simulink model "AM"  (R2020a)
settings: Solver=VariableStepAuto  StartTime=0.0  StopTime=10.0  RelTol=1e-3
libraries: dsparch4 x1
settings Model: Creator=Admin  LastModifiedBy=fazal
settings SFSimCC: CustomCodeUndefinedFunction=UseInterfaceOnly

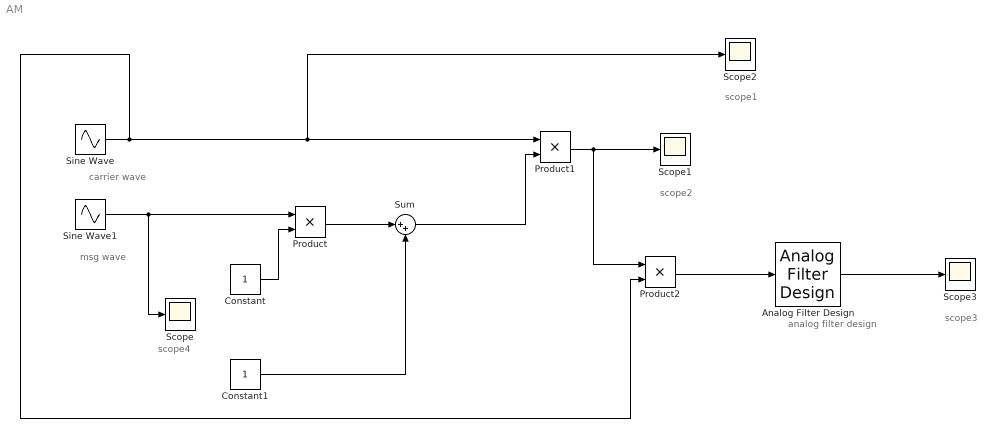
== system AM ==
  note: scope3
  note: scope1
  note: scope2
  note: scope4
  note: analog filter design
  note: msg wave
  note: carrier wave
  Analog Filter Design : dsparch4/Analog Filter Design  method=Butterworth  filttype=Lowpass  N=8  Wlo=30  Whi=80  Rp=2  Rs=40
  Constant : Constant
  Constant1 : Constant
  Product : Product
  Product1 : Product
  Product2 : Product
  Scope{,1..3} (4 alike) : Scope
  Sine Wave : Sin  Amplitude=2  Frequency=2*pi*5  SampleTime=0
  Sine Wave1 : Sin  Frequency=2*pi*1  SampleTime=0
  Sum : Sum  Inputs=|++
  wires:
  Product2/1 -> Analog Filter Design/1
  Analog Filter Design/1 -> Scope3/1
  Sum/1 -> Product1/2
  Product1/1 -> Product2/1, Scope1/1
  Sine Wave1/1 -> Scope/1, Product/1
  Constant/1 -> Product/2
  Product/1 -> Sum/1
  Constant1/1 -> Sum/2
  Sine Wave/1 -> Scope2/1, Product1/1, Product2/2
